simulink model "aes_impl_decrypt_smc"  (R2015b)
settings: Solver=FixedStepDiscrete  SolverMode=SingleTasking  StartTime=0.0  StopTime=1000e-6  RelTol=1e-3
undefined symbols (not defined in the file): a, b, input_sample_rate
libraries: shlslibv1 x3018
(part 8 of 20)

== system aes_impl_decrypt_smc/Round2/Subsystem8/Subsystem1 ==
  In1 : Inport
  In2 : Inport  Port=2
  In3 : Inport  Port=3
  In4 : Inport  Port=4
  Mixcolumn : Subsystem
  Mixcolumn1 : Subsystem
  Mixcolumn2 : Subsystem
  Mixcolumn3 : Subsystem
  Out1 : Outport
  Out2 : Outport  Port=2
  Out3 : Outport  Port=3
  Out4 : Outport  Port=4
  wires:
  Mixcolumn/1(Out1) -> Out1/1
  In4/1 -> Mixcolumn/4(In4), Mixcolumn1/4(In4), Mixcolumn2/4(In4), Mixcolumn3/4(In4)
  Mixcolumn2/1(Out1) -> Out3/1
  Mixcolumn1/1(Out1) -> Out2/1
  In2/1 -> Mixcolumn/2(In2), Mixcolumn1/2(In2), Mixcolumn3/2(In2), Mixcolumn2/2(In2)
  In1/1 -> Mixcolumn2/1(In1), Mixcolumn3/1(In1), Mixcolumn1/1(In1), Mixcolumn/1(In1)
  In3/1 -> Mixcolumn/3(In3), Mixcolumn1/3(In3), Mixcolumn3/3(In3), Mixcolumn2/3(In3)
  Mixcolumn3/1(Out1) -> Out4/1

== system aes_impl_decrypt_smc/Round2/Subsystem8/Subsystem2 ==
  In1 : Inport
  In2 : Inport  Port=2
  In3 : Inport  Port=3
  In4 : Inport  Port=4
  Mixcolumn : Subsystem
  Mixcolumn1 : Subsystem
  Mixcolumn2 : Subsystem
  Mixcolumn3 : Subsystem
  Out1 : Outport
  Out2 : Outport  Port=2
  Out3 : Outport  Port=3
  Out4 : Outport  Port=4
  wires:
  Mixcolumn/1(Out1) -> Out1/1
  In4/1 -> Mixcolumn/4(In4), Mixcolumn1/4(In4), Mixcolumn2/4(In4), Mixcolumn3/4(In4)
  Mixcolumn2/1(Out1) -> Out3/1
  Mixcolumn1/1(Out1) -> Out2/1
  In2/1 -> Mixcolumn/2(In2), Mixcolumn1/2(In2), Mixcolumn3/2(In2), Mixcolumn2/2(In2)
  In1/1 -> Mixcolumn2/1(In1), Mixcolumn3/1(In1), Mixcolumn1/1(In1), Mixcolumn/1(In1)
  In3/1 -> Mixcolumn/3(In3), Mixcolumn1/3(In3), Mixcolumn3/3(In3), Mixcolumn2/3(In3)
  Mixcolumn3/1(Out1) -> Out4/1

== system aes_impl_decrypt_smc/Round2/Subsystem8/Subsystem3 ==
  In1 : Inport
  In2 : Inport  Port=2
  In3 : Inport  Port=3
  In4 : Inport  Port=4
  Mixcolumn : Subsystem
  Mixcolumn1 : Subsystem
  Mixcolumn2 : Subsystem
  Mixcolumn3 : Subsystem
  Out1 : Outport
  Out2 : Outport  Port=2
  Out3 : Outport  Port=3
  Out4 : Outport  Port=4
  wires:
  Mixcolumn/1(Out1) -> Out1/1
  In4/1 -> Mixcolumn/4(In4), Mixcolumn1/4(In4), Mixcolumn2/4(In4), Mixcolumn3/4(In4)
  Mixcolumn2/1(Out1) -> Out3/1
  Mixcolumn1/1(Out1) -> Out2/1
  In2/1 -> Mixcolumn/2(In2), Mixcolumn1/2(In2), Mixcolumn3/2(In2), Mixcolumn2/2(In2)
  In1/1 -> Mixcolumn2/1(In1), Mixcolumn3/1(In1), Mixcolumn1/1(In1), Mixcolumn/1(In1)
  In3/1 -> Mixcolumn/3(In3), Mixcolumn1/3(In3), Mixcolumn3/3(In3), Mixcolumn2/3(In3)
  Mixcolumn3/1(Out1) -> Out4/1

== system aes_impl_decrypt_smc/Round2/Subsystem8/Subsystem4 ==
  In1 : Inport
  In2 : Inport  Port=2
  In3 : Inport  Port=3
  In4 : Inport  Port=4
  ROM{1..4} (4 alike) : shlslibv1/Memories/ROM  syn_rom_vec=sbox  syn_rom_auto_wl=on  syn_out_wl=8  syn_out_fl=0  syn_out_dt=unsigned  syn_out_sat=on  syn_out_rnd=on  syn_en_port=off  synBlockType=primitive  synLatency=1  synBlockId=62  syn_dual_port=off
  Out1 : Outport
  Out2 : Outport  Port=2
  Out3 : Outport  Port=3
  Out4 : Outport  Port=4
  wires:
  In1/1 -> ROM4/1
  In4/1 -> ROM3/1
  In3/1 -> ROM2/1
  ROM4/1 -> Out1/1
  ROM1/1 -> Out2/1
  ROM2/1 -> Out3/1
  ROM3/1 -> Out4/1
  In2/1 -> ROM1/1

== system aes_impl_decrypt_smc/Round2/Subsystem8/Subsystem5 ==
  In1 : Inport
  In2 : Inport  Port=2
  In3 : Inport  Port=3
  In4 : Inport  Port=4
  ROM{1..4} (4 alike) : shlslibv1/Memories/ROM  syn_rom_vec=sbox  syn_rom_auto_wl=on  syn_out_wl=8  syn_out_fl=0  syn_out_dt=unsigned  syn_out_sat=on  syn_out_rnd=on  syn_en_port=off  synBlockType=primitive  synLatency=1  synBlockId=62  syn_dual_port=off
  Out1 : Outport
  Out2 : Outport  Port=2
  Out3 : Outport  Port=3
  Out4 : Outport  Port=4
  wires:
  In1/1 -> ROM4/1
  In4/1 -> ROM3/1
  In3/1 -> ROM2/1
  ROM4/1 -> Out1/1
  ROM1/1 -> Out2/1
  ROM2/1 -> Out3/1
  ROM3/1 -> Out4/1
  In2/1 -> ROM1/1

== system aes_impl_decrypt_smc/Round2/Subsystem8/Subsystem6 ==
  In1 : Inport
  In2 : Inport  Port=2
  In3 : Inport  Port=3
  In4 : Inport  Port=4
  ROM{1..4} (4 alike) : shlslibv1/Memories/ROM  syn_rom_vec=sbox  syn_rom_auto_wl=on  syn_out_wl=8  syn_out_fl=0  syn_out_dt=unsigned  syn_out_sat=on  syn_out_rnd=on  syn_en_port=off  synBlockType=primitive  synLatency=1  synBlockId=62  syn_dual_port=off
  Out1 : Outport
  Out2 : Outport  Port=2
  Out3 : Outport  Port=3
  Out4 : Outport  Port=4
  wires:
  In1/1 -> ROM4/1
  In4/1 -> ROM3/1
  In3/1 -> ROM2/1
  ROM4/1 -> Out1/1
  ROM1/1 -> Out2/1
  ROM2/1 -> Out3/1
  ROM3/1 -> Out4/1
  In2/1 -> ROM1/1

== system aes_impl_decrypt_smc/Round2/Subsystem8/Subsystem7 ==
  In1 : Inport
  In2 : Inport  Port=2
  In3 : Inport  Port=3
  In4 : Inport  Port=4
  ROM{1..4} (4 alike) : shlslibv1/Memories/ROM  syn_rom_vec=sbox  syn_rom_auto_wl=on  syn_out_wl=8  syn_out_fl=0  syn_out_dt=unsigned  syn_out_sat=on  syn_out_rnd=on  syn_en_port=off  synBlockType=primitive  synLatency=1  synBlockId=62  syn_dual_port=off
  Out1 : Outport
  Out2 : Outport  Port=2
  Out3 : Outport  Port=3
  Out4 : Outport  Port=4
  wires:
  In1/1 -> ROM4/1
  In4/1 -> ROM3/1
  In3/1 -> ROM2/1
  ROM4/1 -> Out1/1
  ROM1/1 -> Out2/1
  ROM2/1 -> Out3/1
  ROM3/1 -> Out4/1
  In2/1 -> ROM1/1

== system aes_impl_decrypt_smc/Round20/Subsystem8/Subsystem ==
  In1 : Inport
  In2 : Inport  Port=2
  In3 : Inport  Port=3
  In4 : Inport  Port=4
  In5 : Inport  Port=5
  In6 : Inport  Port=6
  In7 : Inport  Port=7
  In8 : Inport  Port=8
  In9 : Inport  Port=9
  In10 : Inport  Port=10
  In11 : Inport  Port=11
  In12 : Inport  Port=12
  In13 : Inport  Port=13
  In14 : Inport  Port=14
  In15 : Inport  Port=15
  In16 : Inport  Port=16
  Out1 : Outport
  Out2 : Outport  Port=2
  Out3 : Outport  Port=3
  Out4 : Outport  Port=4
  Out5 : Outport  Port=5
  Out6 : Outport  Port=6
  Out7 : Outport  Port=7
  Out8 : Outport  Port=8
  Out9 : Outport  Port=9
  Out10 : Outport  Port=10
  Out11 : Outport  Port=11
  Out12 : Outport  Port=12
  Out13 : Outport  Port=13
  Out14 : Outport  Port=14
  Out15 : Outport  Port=15
  Out16 : Outport  Port=16
  wires:
  In1/1 -> Out1/1
  In5/1 -> Out5/1
  In9/1 -> Out9/1
  In13/1 -> Out13/1
  In2/1 -> Out6/1
  In3/1 -> Out11/1
  In4/1 -> Out16/1
  In6/1 -> Out10/1
  In7/1 -> Out15/1
  In8/1 -> Out4/1
  In10/1 -> Out14/1
  In11/1 -> Out3/1
  In12/1 -> Out8/1
  In14/1 -> Out2/1
  In15/1 -> Out7/1
  In16/1 -> Out12/1

== system aes_impl_decrypt_smc/Round20/Subsystem8/Subsystem1 ==
  In1 : Inport
  In2 : Inport  Port=2
  In3 : Inport  Port=3
  In4 : Inport  Port=4
  ROM{1..4} (4 alike) : shlslibv1/Memories/ROM  syn_rom_vec=isbox  syn_rom_auto_wl=on  syn_out_wl=8  syn_out_fl=0  syn_out_dt=unsigned  syn_out_sat=on  syn_out_rnd=on  syn_en_port=off  synBlockType=primitive  synLatency=1  synBlockId=62  syn_dual_port=off
  Out1 : Outport
  Out2 : Outport  Port=2
  Out3 : Outport  Port=3
  Out4 : Outport  Port=4
  wires:
  In1/1 -> ROM4/1
  In4/1 -> ROM3/1
  In3/1 -> ROM2/1
  ROM4/1 -> Out1/1
  ROM1/1 -> Out2/1
  ROM2/1 -> Out3/1
  ROM3/1 -> Out4/1
  In2/1 -> ROM1/1

== system aes_impl_decrypt_smc/Round20/Subsystem8/Subsystem2 ==
  In1 : Inport
  In2 : Inport  Port=2
  In3 : Inport  Port=3
  In4 : Inport  Port=4
  ROM{1..4} (4 alike) : shlslibv1/Memories/ROM  syn_rom_vec=isbox  syn_rom_auto_wl=on  syn_out_wl=8  syn_out_fl=0  syn_out_dt=unsigned  syn_out_sat=on  syn_out_rnd=on  syn_en_port=off  synBlockType=primitive  synLatency=1  synBlockId=62  syn_dual_port=off
  Out1 : Outport
  Out2 : Outport  Port=2
  Out3 : Outport  Port=3
  Out4 : Outport  Port=4
  wires:
  In1/1 -> ROM4/1
  In4/1 -> ROM3/1
  In3/1 -> ROM2/1
  ROM4/1 -> Out1/1
  ROM1/1 -> Out2/1
  ROM2/1 -> Out3/1
  ROM3/1 -> Out4/1
  In2/1 -> ROM1/1

== system aes_impl_decrypt_smc/Round20/Subsystem8/Subsystem3 ==
  In1 : Inport
  In2 : Inport  Port=2
  In3 : Inport  Port=3
  In4 : Inport  Port=4
  ROM{1..4} (4 alike) : shlslibv1/Memories/ROM  syn_rom_vec=isbox  syn_rom_auto_wl=on  syn_out_wl=8  syn_out_fl=0  syn_out_dt=unsigned  syn_out_sat=on  syn_out_rnd=on  syn_en_port=off  synBlockType=primitive  synLatency=1  synBlockId=62  syn_dual_port=off
  Out1 : Outport
  Out2 : Outport  Port=2
  Out3 : Outport  Port=3
  Out4 : Outport  Port=4
  wires:
  In1/1 -> ROM4/1
  In4/1 -> ROM3/1
  In3/1 -> ROM2/1
  ROM4/1 -> Out1/1
  ROM1/1 -> Out2/1
  ROM2/1 -> Out3/1
  ROM3/1 -> Out4/1
  In2/1 -> ROM1/1

== system aes_impl_decrypt_smc/Round20/Subsystem8/Subsystem4 ==
  In1 : Inport
  In2 : Inport  Port=2
  In3 : Inport  Port=3
  In4 : Inport  Port=4
  ROM{1..4} (4 alike) : shlslibv1/Memories/ROM  syn_rom_vec=isbox  syn_rom_auto_wl=on  syn_out_wl=8  syn_out_fl=0  syn_out_dt=unsigned  syn_out_sat=on  syn_out_rnd=on  syn_en_port=off  synBlockType=primitive  synLatency=1  synBlockId=62  syn_dual_port=off
  Out1 : Outport
  Out2 : Outport  Port=2
  Out3 : Outport  Port=3
  Out4 : Outport  Port=4
  wires:
  In1/1 -> ROM4/1
  In4/1 -> ROM3/1
  In3/1 -> ROM2/1
  ROM4/1 -> Out1/1
  ROM1/1 -> Out2/1
  ROM2/1 -> Out3/1
  ROM3/1 -> Out4/1
  In2/1 -> ROM1/1

== system aes_impl_decrypt_smc/Round20/Subsystem8/Subsystem5 ==
  In17 : Inport
  In18 : Inport  Port=2
  In19 : Inport  Port=3
  In20 : Inport  Port=4
  Mixcolumn : Subsystem
  Mixcolumn1 : Subsystem
  Mixcolumn2 : Subsystem
  Mixcolumn3 : Subsystem
  Out17 : Outport
  Out18 : Outport  Port=2
  Out19 : Outport  Port=3
  Out20 : Outport  Port=4
  wires:
  Mixcolumn3/1(Out1) -> Out20/1
  In20/1 -> Mixcolumn3/4(In4), Mixcolumn2/4(In4), Mixcolumn1/4(In4), Mixcolumn/4(In4)
  In17/1 -> Mixcolumn/1(In1), Mixcolumn1/1(In1), Mixcolumn3/1(In1), Mixcolumn2/1(In1)
  In19/1 -> Mixcolumn1/3(In3), Mixcolumn/3(In3), Mixcolumn3/3(In3), Mixcolumn2/3(In3)
  Mixcolumn1/1(Out1) -> Out18/1
  Mixcolumn/1(Out1) -> Out17/1
  In18/1 -> Mixcolumn1/2(In2), Mixcolumn/2(In2), Mixcolumn3/2(In2), Mixcolumn2/2(In2)
  Mixcolumn2/1(Out1) -> Out19/1

== system aes_impl_decrypt_smc/Round20/Subsystem8/Subsystem6 ==
  In17 : Inport
  In18 : Inport  Port=2
  In19 : Inport  Port=3
  In20 : Inport  Port=4
  Mixcolumn : Subsystem
  Mixcolumn1 : Subsystem
  Mixcolumn2 : Subsystem
  Mixcolumn3 : Subsystem
  Out17 : Outport
  Out18 : Outport  Port=2
  Out19 : Outport  Port=3
  Out20 : Outport  Port=4
  wires:
  Mixcolumn3/1(Out1) -> Out20/1
  In20/1 -> Mixcolumn3/4(In4), Mixcolumn2/4(In4), Mixcolumn1/4(In4), Mixcolumn/4(In4)
  In17/1 -> Mixcolumn/1(In1), Mixcolumn1/1(In1), Mixcolumn3/1(In1), Mixcolumn2/1(In1)
  In19/1 -> Mixcolumn1/3(In3), Mixcolumn/3(In3), Mixcolumn3/3(In3), Mixcolumn2/3(In3)
  Mixcolumn1/1(Out1) -> Out18/1
  Mixcolumn/1(Out1) -> Out17/1
  In18/1 -> Mixcolumn1/2(In2), Mixcolumn/2(In2), Mixcolumn3/2(In2), Mixcolumn2/2(In2)
  Mixcolumn2/1(Out1) -> Out19/1

== system aes_impl_decrypt_smc/Round20/Subsystem8/Subsystem7 ==
  In17 : Inport
  In18 : Inport  Port=2
  In19 : Inport  Port=3
  In20 : Inport  Port=4
  Mixcolumn : Subsystem
  Mixcolumn1 : Subsystem
  Mixcolumn2 : Subsystem
  Mixcolumn3 : Subsystem
  Out17 : Outport
  Out18 : Outport  Port=2
  Out19 : Outport  Port=3
  Out20 : Outport  Port=4
  wires:
  Mixcolumn3/1(Out1) -> Out20/1
  In20/1 -> Mixcolumn3/4(In4), Mixcolumn2/4(In4), Mixcolumn1/4(In4), Mixcolumn/4(In4)
  In17/1 -> Mixcolumn/1(In1), Mixcolumn1/1(In1), Mixcolumn3/1(In1), Mixcolumn2/1(In1)
  In19/1 -> Mixcolumn1/3(In3), Mixcolumn/3(In3), Mixcolumn3/3(In3), Mixcolumn2/3(In3)
  Mixcolumn1/1(Out1) -> Out18/1
  Mixcolumn/1(Out1) -> Out17/1
  In18/1 -> Mixcolumn1/2(In2), Mixcolumn/2(In2), Mixcolumn3/2(In2), Mixcolumn2/2(In2)
  Mixcolumn2/1(Out1) -> Out19/1

== system aes_impl_decrypt_smc/Round20/Subsystem8/Subsystem8 ==
  In17 : Inport
  In18 : Inport  Port=2
  In19 : Inport  Port=3
  In20 : Inport  Port=4
  Mixcolumn : Subsystem
  Mixcolumn1 : Subsystem
  Mixcolumn2 : Subsystem
  Mixcolumn3 : Subsystem
  Out17 : Outport
  Out18 : Outport  Port=2
  Out19 : Outport  Port=3
  Out20 : Outport  Port=4
  wires:
  Mixcolumn3/1(Out1) -> Out20/1
  In20/1 -> Mixcolumn3/4(In4), Mixcolumn2/4(In4), Mixcolumn1/4(In4), Mixcolumn/4(In4)
  In17/1 -> Mixcolumn/1(In1), Mixcolumn1/1(In1), Mixcolumn3/1(In1), Mixcolumn2/1(In1)
  In19/1 -> Mixcolumn1/3(In3), Mixcolumn/3(In3), Mixcolumn3/3(In3), Mixcolumn2/3(In3)
  Mixcolumn1/1(Out1) -> Out18/1
  Mixcolumn/1(Out1) -> Out17/1
  In18/1 -> Mixcolumn1/2(In2), Mixcolumn/2(In2), Mixcolumn3/2(In2), Mixcolumn2/2(In2)
  Mixcolumn2/1(Out1) -> Out19/1

== system aes_impl_decrypt_smc/Round3/Key1/Keygen1 ==
  In1 : Inport
  In2 : Inport  Port=2
  In3 : Inport  Port=3
  In4 : Inport  Port=4
  In5 : Inport  Port=5
  In6 : Inport  Port=6
  In7 : Inport  Port=7
  In8 : Inport  Port=8
  Binary Logic{,1..7} (8 alike) : shlslibv1/Math Functions/Binary Logic  syn_binlog_exp=a^b  synBlockType=primitive  synLatency=0  synBlockId=13
  Constant1 : shlslibv1/Sources/Constant  syn_cst_val=0  syn_cst_format=Specify  syn_cst_wl=8  syn_cst_fl=0  syn_cst_dt=unsigned  syn_cst_rnd=on  syn_cst_st=-1  synBlockType=primitive  synLatency=0  synBlockId=15
  Constant2 : shlslibv1/Sources/Constant  syn_cst_val=0  syn_cst_format=Specify  syn_cst_wl=8  syn_cst_fl=0  syn_cst_dt=unsigned  syn_cst_rnd=on  syn_cst_st=-1  synBlockType=primitive  synLatency=0  synBlockId=15
  Constant3 : shlslibv1/Sources/Constant  syn_cst_val=0  syn_cst_format=Specify  syn_cst_wl=8  syn_cst_fl=0  syn_cst_dt=unsigned  syn_cst_rnd=on  syn_cst_st=-1  synBlockType=primitive  synLatency=0  synBlockId=15
  Constant4 : shlslibv1/Sources/Constant  syn_cst_val=16  syn_cst_format=Specify  syn_cst_wl=8  syn_cst_fl=0  syn_cst_dt=unsigned  syn_cst_rnd=on  syn_cst_st=-1  synBlockType=primitive  synLatency=0  synBlockId=15
  Subsystem4 : Subsystem
  Out1 : Outport
  Out2 : Outport  Port=2
  Out3 : Outport  Port=3
  Out4 : Outport  Port=4
  wires:
  Constant1/1 -> Binary Logic3/2
  Binary Logic3/1 -> Out2/1
  Binary Logic5/1 -> Out3/1
  Binary Logic2/1 -> Out1/1
  Constant3/1 -> Binary Logic7/2
  Binary Logic7/1 -> Out4/1
  Constant2/1 -> Binary Logic5/2
  Subsystem4/3(Out3) -> Binary Logic4/2
  In7/1 -> Subsystem4/2(In2)
  In6/1 -> Subsystem4/1(In1)
  Subsystem4/4(Out4) -> Binary Logic6/2
  Subsystem4/2(Out2) -> Binary Logic1/2
  Subsystem4/1(Out1) -> Binary Logic/2
  In8/1 -> Subsystem4/3(In3)
  In5/1 -> Subsystem4/4(In4)
  In1/1 -> Binary Logic/1
  In2/1 -> Binary Logic1/1
  In3/1 -> Binary Logic4/1
  In4/1 -> Binary Logic6/1
  Constant4/1 -> Binary Logic2/2
  Binary Logic/1 -> Binary Logic2/1
  Binary Logic1/1 -> Binary Logic3/1
  Binary Logic4/1 -> Binary Logic5/1
  Binary Logic6/1 -> Binary Logic7/1

== system aes_impl_decrypt_smc/Round3/Key1/Keygen2 ==
  In1 : Inport
  In2 : Inport  Port=2
  In3 : Inport  Port=3
  In4 : Inport  Port=4
  In5 : Inport  Port=5
  In6 : Inport  Port=6
  In7 : Inport  Port=7
  In8 : Inport  Port=8
  Binary Logic{,1..3} (4 alike) : shlslibv1/Math Functions/Binary Logic  syn_binlog_exp=a^b  synBlockType=primitive  synLatency=0  synBlockId=13
  Out1 : Outport
  Out2 : Outport  Port=2
  Out3 : Outport  Port=3
  Out4 : Outport  Port=4
  wires:
  In6/1 -> Binary Logic1/2
  In2/1 -> Binary Logic1/1
  Binary Logic2/1 -> Out3/1
  In7/1 -> Binary Logic2/2
  In8/1 -> Binary Logic3/2
  Binary Logic1/1 -> Out2/1
  In3/1 -> Binary Logic2/1
  In4/1 -> Binary Logic3/1
  Binary Logic3/1 -> Out4/1
  In1/1 -> Binary Logic/1
  In5/1 -> Binary Logic/2
  Binary Logic/1 -> Out1/1

== system aes_impl_decrypt_smc/Round3/Key1/Keygen3 ==
  In1 : Inport
  In2 : Inport  Port=2
  In3 : Inport  Port=3
  In4 : Inport  Port=4
  In5 : Inport  Port=5
  In6 : Inport  Port=6
  In7 : Inport  Port=7
  In8 : Inport  Port=8
  Binary Logic{,1..3} (4 alike) : shlslibv1/Math Functions/Binary Logic  syn_binlog_exp=a^b  synBlockType=primitive  synLatency=0  synBlockId=13
  Out1 : Outport
  Out2 : Outport  Port=2
  Out3 : Outport  Port=3
  Out4 : Outport  Port=4
  wires:
  In6/1 -> Binary Logic1/2
  In2/1 -> Binary Logic1/1
  Binary Logic2/1 -> Out3/1
  In7/1 -> Binary Logic2/2
  In8/1 -> Binary Logic3/2
  Binary Logic1/1 -> Out2/1
  In3/1 -> Binary Logic2/1
  In4/1 -> Binary Logic3/1
  Binary Logic3/1 -> Out4/1
  In1/1 -> Binary Logic/1
  In5/1 -> Binary Logic/2
  Binary Logic/1 -> Out1/1

== system aes_impl_decrypt_smc/Round3/Key1/Keygen4 ==
  In1 : Inport
  In2 : Inport  Port=2
  In3 : Inport  Port=3
  In4 : Inport  Port=4
  In5 : Inport  Port=5
  In6 : Inport  Port=6
  In7 : Inport  Port=7
  In8 : Inport  Port=8
  Binary Logic{,1..3} (4 alike) : shlslibv1/Math Functions/Binary Logic  syn_binlog_exp=a^b  synBlockType=primitive  synLatency=0  synBlockId=13
  Out1 : Outport
  Out2 : Outport  Port=2
  Out3 : Outport  Port=3
  Out4 : Outport  Port=4
  wires:
  In6/1 -> Binary Logic1/2
  In2/1 -> Binary Logic1/1
  Binary Logic2/1 -> Out3/1
  In7/1 -> Binary Logic2/2
  In8/1 -> Binary Logic3/2
  Binary Logic1/1 -> Out2/1
  In3/1 -> Binary Logic2/1
  In4/1 -> Binary Logic3/1
  Binary Logic3/1 -> Out4/1
  In1/1 -> Binary Logic/1
  In5/1 -> Binary Logic/2
  Binary Logic/1 -> Out1/1

== system aes_impl_decrypt_smc/Round3/Subsystem8/Subsystem ==
  In1 : Inport
  In2 : Inport  Port=2
  In3 : Inport  Port=3
  In4 : Inport  Port=4
  Mixcolumn : Subsystem
  Mixcolumn1 : Subsystem
  Mixcolumn2 : Subsystem
  Mixcolumn3 : Subsystem
  Out1 : Outport
  Out2 : Outport  Port=2
  Out3 : Outport  Port=3
  Out4 : Outport  Port=4
  wires:
  Mixcolumn/1(Out1) -> Out1/1
  In4/1 -> Mixcolumn/4(In4), Mixcolumn1/4(In4), Mixcolumn2/4(In4), Mixcolumn3/4(In4)
  Mixcolumn2/1(Out1) -> Out3/1
  Mixcolumn1/1(Out1) -> Out2/1
  In2/1 -> Mixcolumn/2(In2), Mixcolumn1/2(In2), Mixcolumn3/2(In2), Mixcolumn2/2(In2)
  In1/1 -> Mixcolumn2/1(In1), Mixcolumn3/1(In1), Mixcolumn1/1(In1), Mixcolumn/1(In1)
  In3/1 -> Mixcolumn/3(In3), Mixcolumn1/3(In3), Mixcolumn3/3(In3), Mixcolumn2/3(In3)
  Mixcolumn3/1(Out1) -> Out4/1

== system aes_impl_decrypt_smc/Round3/Subsystem8/Subsystem1 ==
  In1 : Inport
  In2 : Inport  Port=2
  In3 : Inport  Port=3
  In4 : Inport  Port=4
  Mixcolumn : Subsystem
  Mixcolumn1 : Subsystem
  Mixcolumn2 : Subsystem
  Mixcolumn3 : Subsystem
  Out1 : Outport
  Out2 : Outport  Port=2
  Out3 : Outport  Port=3
  Out4 : Outport  Port=4
  wires:
  Mixcolumn/1(Out1) -> Out1/1
  In4/1 -> Mixcolumn/4(In4), Mixcolumn1/4(In4), Mixcolumn2/4(In4), Mixcolumn3/4(In4)
  Mixcolumn2/1(Out1) -> Out3/1
  Mixcolumn1/1(Out1) -> Out2/1
  In2/1 -> Mixcolumn/2(In2), Mixcolumn1/2(In2), Mixcolumn3/2(In2), Mixcolumn2/2(In2)
  In1/1 -> Mixcolumn2/1(In1), Mixcolumn3/1(In1), Mixcolumn1/1(In1), Mixcolumn/1(In1)
  In3/1 -> Mixcolumn/3(In3), Mixcolumn1/3(In3), Mixcolumn3/3(In3), Mixcolumn2/3(In3)
  Mixcolumn3/1(Out1) -> Out4/1

== system aes_impl_decrypt_smc/Round3/Subsystem8/Subsystem2 ==
  In1 : Inport
  In2 : Inport  Port=2
  In3 : Inport  Port=3
  In4 : Inport  Port=4
  Mixcolumn : Subsystem
  Mixcolumn1 : Subsystem
  Mixcolumn2 : Subsystem
  Mixcolumn3 : Subsystem
  Out1 : Outport
  Out2 : Outport  Port=2
  Out3 : Outport  Port=3
  Out4 : Outport  Port=4
  wires:
  Mixcolumn/1(Out1) -> Out1/1
  In4/1 -> Mixcolumn/4(In4), Mixcolumn1/4(In4), Mixcolumn2/4(In4), Mixcolumn3/4(In4)
  Mixcolumn2/1(Out1) -> Out3/1
  Mixcolumn1/1(Out1) -> Out2/1
  In2/1 -> Mixcolumn/2(In2), Mixcolumn1/2(In2), Mixcolumn3/2(In2), Mixcolumn2/2(In2)
  In1/1 -> Mixcolumn2/1(In1), Mixcolumn3/1(In1), Mixcolumn1/1(In1), Mixcolumn/1(In1)
  In3/1 -> Mixcolumn/3(In3), Mixcolumn1/3(In3), Mixcolumn3/3(In3), Mixcolumn2/3(In3)
  Mixcolumn3/1(Out1) -> Out4/1

== system aes_impl_decrypt_smc/Round3/Subsystem8/Subsystem3 ==
  In1 : Inport
  In2 : Inport  Port=2
  In3 : Inport  Port=3
  In4 : Inport  Port=4
  Mixcolumn : Subsystem
  Mixcolumn1 : Subsystem
  Mixcolumn2 : Subsystem
  Mixcolumn3 : Subsystem
  Out1 : Outport
  Out2 : Outport  Port=2
  Out3 : Outport  Port=3
  Out4 : Outport  Port=4
  wires:
  Mixcolumn/1(Out1) -> Out1/1
  In4/1 -> Mixcolumn/4(In4), Mixcolumn1/4(In4), Mixcolumn2/4(In4), Mixcolumn3/4(In4)
  Mixcolumn2/1(Out1) -> Out3/1
  Mixcolumn1/1(Out1) -> Out2/1
  In2/1 -> Mixcolumn/2(In2), Mixcolumn1/2(In2), Mixcolumn3/2(In2), Mixcolumn2/2(In2)
  In1/1 -> Mixcolumn2/1(In1), Mixcolumn3/1(In1), Mixcolumn1/1(In1), Mixcolumn/1(In1)
  In3/1 -> Mixcolumn/3(In3), Mixcolumn1/3(In3), Mixcolumn3/3(In3), Mixcolumn2/3(In3)
  Mixcolumn3/1(Out1) -> Out4/1

== system aes_impl_decrypt_smc/Round3/Subsystem8/Subsystem4 ==
  In1 : Inport
  In2 : Inport  Port=2
  In3 : Inport  Port=3
  In4 : Inport  Port=4
  ROM{1..4} (4 alike) : shlslibv1/Memories/ROM  syn_rom_vec=sbox  syn_rom_auto_wl=on  syn_out_wl=8  syn_out_fl=0  syn_out_dt=unsigned  syn_out_sat=on  syn_out_rnd=on  syn_en_port=off  synBlockType=primitive  synLatency=1  synBlockId=62  syn_dual_port=off
  Out1 : Outport
  Out2 : Outport  Port=2
  Out3 : Outport  Port=3
  Out4 : Outport  Port=4
  wires:
  In1/1 -> ROM4/1
  In4/1 -> ROM3/1
  In3/1 -> ROM2/1
  ROM4/1 -> Out1/1
  ROM1/1 -> Out2/1
  ROM2/1 -> Out3/1
  ROM3/1 -> Out4/1
  In2/1 -> ROM1/1

== system aes_impl_decrypt_smc/Round3/Subsystem8/Subsystem5 ==
  In1 : Inport
  In2 : Inport  Port=2
  In3 : Inport  Port=3
  In4 : Inport  Port=4
  ROM{1..4} (4 alike) : shlslibv1/Memories/ROM  syn_rom_vec=sbox  syn_rom_auto_wl=on  syn_out_wl=8  syn_out_fl=0  syn_out_dt=unsigned  syn_out_sat=on  syn_out_rnd=on  syn_en_port=off  synBlockType=primitive  synLatency=1  synBlockId=62  syn_dual_port=off
  Out1 : Outport
  Out2 : Outport  Port=2
  Out3 : Outport  Port=3
  Out4 : Outport  Port=4
  wires:
  In1/1 -> ROM4/1
  In4/1 -> ROM3/1
  In3/1 -> ROM2/1
  ROM4/1 -> Out1/1
  ROM1/1 -> Out2/1
  ROM2/1 -> Out3/1
  ROM3/1 -> Out4/1
  In2/1 -> ROM1/1

== system aes_impl_decrypt_smc/Round3/Subsystem8/Subsystem6 ==
  In1 : Inport
  In2 : Inport  Port=2
  In3 : Inport  Port=3
  In4 : Inport  Port=4
  ROM{1..4} (4 alike) : shlslibv1/Memories/ROM  syn_rom_vec=sbox  syn_rom_auto_wl=on  syn_out_wl=8  syn_out_fl=0  syn_out_dt=unsigned  syn_out_sat=on  syn_out_rnd=on  syn_en_port=off  synBlockType=primitive  synLatency=1  synBlockId=62  syn_dual_port=off
  Out1 : Outport
  Out2 : Outport  Port=2
  Out3 : Outport  Port=3
  Out4 : Outport  Port=4
  wires:
  In1/1 -> ROM4/1
  In4/1 -> ROM3/1
  In3/1 -> ROM2/1
  ROM4/1 -> Out1/1
  ROM1/1 -> Out2/1
  ROM2/1 -> Out3/1
  ROM3/1 -> Out4/1
  In2/1 -> ROM1/1

== system aes_impl_decrypt_smc/Round3/Subsystem8/Subsystem7 ==
  In1 : Inport
  In2 : Inport  Port=2
  In3 : Inport  Port=3
  In4 : Inport  Port=4
  ROM{1..4} (4 alike) : shlslibv1/Memories/ROM  syn_rom_vec=sbox  syn_rom_auto_wl=on  syn_out_wl=8  syn_out_fl=0  syn_out_dt=unsigned  syn_out_sat=on  syn_out_rnd=on  syn_en_port=off  synBlockType=primitive  synLatency=1  synBlockId=62  syn_dual_port=off
  Out1 : Outport
  Out2 : Outport  Port=2
  Out3 : Outport  Port=3
  Out4 : Outport  Port=4
  wires:
  In1/1 -> ROM4/1
  In4/1 -> ROM3/1
  In3/1 -> ROM2/1
  ROM4/1 -> Out1/1
  ROM1/1 -> Out2/1
  ROM2/1 -> Out3/1
  ROM3/1 -> Out4/1
  In2/1 -> ROM1/1

== system aes_impl_decrypt_smc/Round4/Key1/Keygen1 ==
  In1 : Inport
  In2 : Inport  Port=2
  In3 : Inport  Port=3
  In4 : Inport  Port=4
  In5 : Inport  Port=5
  In6 : Inport  Port=6
  In7 : Inport  Port=7
  In8 : Inport  Port=8
  Binary Logic{,1..7} (8 alike) : shlslibv1/Math Functions/Binary Logic  syn_binlog_exp=a^b  synBlockType=primitive  synLatency=0  synBlockId=13
  Constant1 : shlslibv1/Sources/Constant  syn_cst_val=0  syn_cst_format=Specify  syn_cst_wl=8  syn_cst_fl=0  syn_cst_dt=unsigned  syn_cst_rnd=on  syn_cst_st=-1  synBlockType=primitive  synLatency=0  synBlockId=15
  Constant2 : shlslibv1/Sources/Constant  syn_cst_val=0  syn_cst_format=Specify  syn_cst_wl=8  syn_cst_fl=0  syn_cst_dt=unsigned  syn_cst_rnd=on  syn_cst_st=-1  synBlockType=primitive  synLatency=0  synBlockId=15
  Constant3 : shlslibv1/Sources/Constant  syn_cst_val=0  syn_cst_format=Specify  syn_cst_wl=8  syn_cst_fl=0  syn_cst_dt=unsigned  syn_cst_rnd=on  syn_cst_st=-1  synBlockType=primitive  synLatency=0  synBlockId=15
  Constant4 : shlslibv1/Sources/Constant  syn_cst_val=4  syn_cst_format=Specify  syn_cst_wl=8  syn_cst_fl=0  syn_cst_dt=unsigned  syn_cst_rnd=on  syn_cst_st=-1  synBlockType=primitive  synLatency=0  synBlockId=15
  Subsystem4 : Subsystem
  Out1 : Outport
  Out2 : Outport  Port=2
  Out3 : Outport  Port=3
  Out4 : Outport  Port=4
  wires:
  Constant1/1 -> Binary Logic3/2
  Binary Logic3/1 -> Out2/1
  Binary Logic5/1 -> Out3/1
  Binary Logic2/1 -> Out1/1
  Constant3/1 -> Binary Logic7/2
  Binary Logic7/1 -> Out4/1
  Constant2/1 -> Binary Logic5/2
  Subsystem4/3(Out3) -> Binary Logic4/2
  In7/1 -> Subsystem4/2(In2)
  In6/1 -> Subsystem4/1(In1)
  Subsystem4/4(Out4) -> Binary Logic6/2
  Subsystem4/2(Out2) -> Binary Logic1/2
  Subsystem4/1(Out1) -> Binary Logic/2
  In8/1 -> Subsystem4/3(In3)
  In5/1 -> Subsystem4/4(In4)
  In1/1 -> Binary Logic/1
  In2/1 -> Binary Logic1/1
  In3/1 -> Binary Logic4/1
  In4/1 -> Binary Logic6/1
  Constant4/1 -> Binary Logic2/2
  Binary Logic/1 -> Binary Logic2/1
  Binary Logic1/1 -> Binary Logic3/1
  Binary Logic4/1 -> Binary Logic5/1
  Binary Logic6/1 -> Binary Logic7/1

== system aes_impl_decrypt_smc/Round4/Key1/Keygen2 ==
  In1 : Inport
  In2 : Inport  Port=2
  In3 : Inport  Port=3
  In4 : Inport  Port=4
  In5 : Inport  Port=5
  In6 : Inport  Port=6
  In7 : Inport  Port=7
  In8 : Inport  Port=8
  Binary Logic{,1..3} (4 alike) : shlslibv1/Math Functions/Binary Logic  syn_binlog_exp=a^b  synBlockType=primitive  synLatency=0  synBlockId=13
  Out1 : Outport
  Out2 : Outport  Port=2
  Out3 : Outport  Port=3
  Out4 : Outport  Port=4
  wires:
  In6/1 -> Binary Logic1/2
  In2/1 -> Binary Logic1/1
  Binary Logic2/1 -> Out3/1
  In7/1 -> Binary Logic2/2
  In8/1 -> Binary Logic3/2
  Binary Logic1/1 -> Out2/1
  In3/1 -> Binary Logic2/1
  In4/1 -> Binary Logic3/1
  Binary Logic3/1 -> Out4/1
  In1/1 -> Binary Logic/1
  In5/1 -> Binary Logic/2
  Binary Logic/1 -> Out1/1

== system aes_impl_decrypt_smc/Round4/Key1/Keygen3 ==
  In1 : Inport
  In2 : Inport  Port=2
  In3 : Inport  Port=3
  In4 : Inport  Port=4
  In5 : Inport  Port=5
  In6 : Inport  Port=6
  In7 : Inport  Port=7
  In8 : Inport  Port=8
  Binary Logic{,1..3} (4 alike) : shlslibv1/Math Functions/Binary Logic  syn_binlog_exp=a^b  synBlockType=primitive  synLatency=0  synBlockId=13
  Out1 : Outport
  Out2 : Outport  Port=2
  Out3 : Outport  Port=3
  Out4 : Outport  Port=4
  wires:
  In6/1 -> Binary Logic1/2
  In2/1 -> Binary Logic1/1
  Binary Logic2/1 -> Out3/1
  In7/1 -> Binary Logic2/2
  In8/1 -> Binary Logic3/2
  Binary Logic1/1 -> Out2/1
  In3/1 -> Binary Logic2/1
  In4/1 -> Binary Logic3/1
  Binary Logic3/1 -> Out4/1
  In1/1 -> Binary Logic/1
  In5/1 -> Binary Logic/2
  Binary Logic/1 -> Out1/1

== system aes_impl_decrypt_smc/Round4/Key1/Keygen4 ==
  In1 : Inport
  In2 : Inport  Port=2
  In3 : Inport  Port=3
  In4 : Inport  Port=4
  In5 : Inport  Port=5
  In6 : Inport  Port=6
  In7 : Inport  Port=7
  In8 : Inport  Port=8
  Binary Logic{,1..3} (4 alike) : shlslibv1/Math Functions/Binary Logic  syn_binlog_exp=a^b  synBlockType=primitive  synLatency=0  synBlockId=13
  Out1 : Outport
  Out2 : Outport  Port=2
  Out3 : Outport  Port=3
  Out4 : Outport  Port=4
  wires:
  In6/1 -> Binary Logic1/2
  In2/1 -> Binary Logic1/1
  Binary Logic2/1 -> Out3/1
  In7/1 -> Binary Logic2/2
  In8/1 -> Binary Logic3/2
  Binary Logic1/1 -> Out2/1
  In3/1 -> Binary Logic2/1
  In4/1 -> Binary Logic3/1
  Binary Logic3/1 -> Out4/1
  In1/1 -> Binary Logic/1
  In5/1 -> Binary Logic/2
  Binary Logic/1 -> Out1/1

== system aes_impl_decrypt_smc/Round4/Subsystem8/Subsystem ==
  In1 : Inport
  In2 : Inport  Port=2
  In3 : Inport  Port=3
  In4 : Inport  Port=4
  Mixcolumn : Subsystem
  Mixcolumn1 : Subsystem
  Mixcolumn2 : Subsystem
  Mixcolumn3 : Subsystem
  Out1 : Outport
  Out2 : Outport  Port=2
  Out3 : Outport  Port=3
  Out4 : Outport  Port=4
  wires:
  Mixcolumn/1(Out1) -> Out1/1
  In4/1 -> Mixcolumn/4(In4), Mixcolumn1/4(In4), Mixcolumn2/4(In4), Mixcolumn3/4(In4)
  Mixcolumn2/1(Out1) -> Out3/1
  Mixcolumn1/1(Out1) -> Out2/1
  In2/1 -> Mixcolumn/2(In2), Mixcolumn1/2(In2), Mixcolumn3/2(In2), Mixcolumn2/2(In2)
  In1/1 -> Mixcolumn2/1(In1), Mixcolumn3/1(In1), Mixcolumn1/1(In1), Mixcolumn/1(In1)
  In3/1 -> Mixcolumn/3(In3), Mixcolumn1/3(In3), Mixcolumn3/3(In3), Mixcolumn2/3(In3)
  Mixcolumn3/1(Out1) -> Out4/1

== system aes_impl_decrypt_smc/Round4/Subsystem8/Subsystem1 ==
  In1 : Inport
  In2 : Inport  Port=2
  In3 : Inport  Port=3
  In4 : Inport  Port=4
  Mixcolumn : Subsystem
  Mixcolumn1 : Subsystem
  Mixcolumn2 : Subsystem
  Mixcolumn3 : Subsystem
  Out1 : Outport
  Out2 : Outport  Port=2
  Out3 : Outport  Port=3
  Out4 : Outport  Port=4
  wires:
  Mixcolumn/1(Out1) -> Out1/1
  In4/1 -> Mixcolumn/4(In4), Mixcolumn1/4(In4), Mixcolumn2/4(In4), Mixcolumn3/4(In4)
  Mixcolumn2/1(Out1) -> Out3/1
  Mixcolumn1/1(Out1) -> Out2/1
  In2/1 -> Mixcolumn/2(In2), Mixcolumn1/2(In2), Mixcolumn3/2(In2), Mixcolumn2/2(In2)
  In1/1 -> Mixcolumn2/1(In1), Mixcolumn3/1(In1), Mixcolumn1/1(In1), Mixcolumn/1(In1)
  In3/1 -> Mixcolumn/3(In3), Mixcolumn1/3(In3), Mixcolumn3/3(In3), Mixcolumn2/3(In3)
  Mixcolumn3/1(Out1) -> Out4/1

== system aes_impl_decrypt_smc/Round4/Subsystem8/Subsystem2 ==
  In1 : Inport
  In2 : Inport  Port=2
  In3 : Inport  Port=3
  In4 : Inport  Port=4
  Mixcolumn : Subsystem
  Mixcolumn1 : Subsystem
  Mixcolumn2 : Subsystem
  Mixcolumn3 : Subsystem
  Out1 : Outport
  Out2 : Outport  Port=2
  Out3 : Outport  Port=3
  Out4 : Outport  Port=4
  wires:
  Mixcolumn/1(Out1) -> Out1/1
  In4/1 -> Mixcolumn/4(In4), Mixcolumn1/4(In4), Mixcolumn2/4(In4), Mixcolumn3/4(In4)
  Mixcolumn2/1(Out1) -> Out3/1
  Mixcolumn1/1(Out1) -> Out2/1
  In2/1 -> Mixcolumn/2(In2), Mixcolumn1/2(In2), Mixcolumn3/2(In2), Mixcolumn2/2(In2)
  In1/1 -> Mixcolumn2/1(In1), Mixcolumn3/1(In1), Mixcolumn1/1(In1), Mixcolumn/1(In1)
  In3/1 -> Mixcolumn/3(In3), Mixcolumn1/3(In3), Mixcolumn3/3(In3), Mixcolumn2/3(In3)
  Mixcolumn3/1(Out1) -> Out4/1

== system aes_impl_decrypt_smc/Round4/Subsystem8/Subsystem3 ==
  In1 : Inport
  In2 : Inport  Port=2
  In3 : Inport  Port=3
  In4 : Inport  Port=4
  Mixcolumn : Subsystem
  Mixcolumn1 : Subsystem
  Mixcolumn2 : Subsystem
  Mixcolumn3 : Subsystem
  Out1 : Outport
  Out2 : Outport  Port=2
  Out3 : Outport  Port=3
  Out4 : Outport  Port=4
  wires:
  Mixcolumn/1(Out1) -> Out1/1
  In4/1 -> Mixcolumn/4(In4), Mixcolumn1/4(In4), Mixcolumn2/4(In4), Mixcolumn3/4(In4)
  Mixcolumn2/1(Out1) -> Out3/1
  Mixcolumn1/1(Out1) -> Out2/1
  In2/1 -> Mixcolumn/2(In2), Mixcolumn1/2(In2), Mixcolumn3/2(In2), Mixcolumn2/2(In2)
  In1/1 -> Mixcolumn2/1(In1), Mixcolumn3/1(In1), Mixcolumn1/1(In1), Mixcolumn/1(In1)
  In3/1 -> Mixcolumn/3(In3), Mixcolumn1/3(In3), Mixcolumn3/3(In3), Mixcolumn2/3(In3)
  Mixcolumn3/1(Out1) -> Out4/1

== system aes_impl_decrypt_smc/Round4/Subsystem8/Subsystem4 ==
  In1 : Inport
  In2 : Inport  Port=2
  In3 : Inport  Port=3
  In4 : Inport  Port=4
  ROM{1..4} (4 alike) : shlslibv1/Memories/ROM  syn_rom_vec=sbox  syn_rom_auto_wl=on  syn_out_wl=8  syn_out_fl=0  syn_out_dt=unsigned  syn_out_sat=on  syn_out_rnd=on  syn_en_port=off  synBlockType=primitive  synLatency=1  synBlockId=62  syn_dual_port=off
  Out1 : Outport
  Out2 : Outport  Port=2
  Out3 : Outport  Port=3
  Out4 : Outport  Port=4
  wires:
  In1/1 -> ROM4/1
  In4/1 -> ROM3/1
  In3/1 -> ROM2/1
  ROM4/1 -> Out1/1
  ROM1/1 -> Out2/1
  ROM2/1 -> Out3/1
  ROM3/1 -> Out4/1
  In2/1 -> ROM1/1

== system aes_impl_decrypt_smc/Round4/Subsystem8/Subsystem5 ==
  In1 : Inport
  In2 : Inport  Port=2
  In3 : Inport  Port=3
  In4 : Inport  Port=4
  ROM{1..4} (4 alike) : shlslibv1/Memories/ROM  syn_rom_vec=sbox  syn_rom_auto_wl=on  syn_out_wl=8  syn_out_fl=0  syn_out_dt=unsigned  syn_out_sat=on  syn_out_rnd=on  syn_en_port=off  synBlockType=primitive  synLatency=1  synBlockId=62  syn_dual_port=off
  Out1 : Outport
  Out2 : Outport  Port=2
  Out3 : Outport  Port=3
  Out4 : Outport  Port=4
  wires:
  In1/1 -> ROM4/1
  In4/1 -> ROM3/1
  In3/1 -> ROM2/1
  ROM4/1 -> Out1/1
  ROM1/1 -> Out2/1
  ROM2/1 -> Out3/1
  ROM3/1 -> Out4/1
  In2/1 -> ROM1/1

== system aes_impl_decrypt_smc/Round4/Subsystem8/Subsystem6 ==
  In1 : Inport
  In2 : Inport  Port=2
  In3 : Inport  Port=3
  In4 : Inport  Port=4
  ROM{1..4} (4 alike) : shlslibv1/Memories/ROM  syn_rom_vec=sbox  syn_rom_auto_wl=on  syn_out_wl=8  syn_out_fl=0  syn_out_dt=unsigned  syn_out_sat=on  syn_out_rnd=on  syn_en_port=off  synBlockType=primitive  synLatency=1  synBlockId=62  syn_dual_port=off
  Out1 : Outport
  Out2 : Outport  Port=2
  Out3 : Outport  Port=3
  Out4 : Outport  Port=4
  wires:
  In1/1 -> ROM4/1
  In4/1 -> ROM3/1
  In3/1 -> ROM2/1
  ROM4/1 -> Out1/1
  ROM1/1 -> Out2/1
  ROM2/1 -> Out3/1
  ROM3/1 -> Out4/1
  In2/1 -> ROM1/1

== system aes_impl_decrypt_smc/Round4/Subsystem8/Subsystem7 ==
  In1 : Inport
  In2 : Inport  Port=2
  In3 : Inport  Port=3
  In4 : Inport  Port=4
  ROM{1..4} (4 alike) : shlslibv1/Memories/ROM  syn_rom_vec=sbox  syn_rom_auto_wl=on  syn_out_wl=8  syn_out_fl=0  syn_out_dt=unsigned  syn_out_sat=on  syn_out_rnd=on  syn_en_port=off  synBlockType=primitive  synLatency=1  synBlockId=62  syn_dual_port=off
  Out1 : Outport
  Out2 : Outport  Port=2
  Out3 : Outport  Port=3
  Out4 : Outport  Port=4
  wires:
  In1/1 -> ROM4/1
  In4/1 -> ROM3/1
  In3/1 -> ROM2/1
  ROM4/1 -> Out1/1
  ROM1/1 -> Out2/1
  ROM2/1 -> Out3/1
  ROM3/1 -> Out4/1
  In2/1 -> ROM1/1

== system aes_impl_decrypt_smc/Round5/Key1/Keygen1 ==
  In1 : Inport
  In2 : Inport  Port=2
  In3 : Inport  Port=3
  In4 : Inport  Port=4
  In5 : Inport  Port=5
  In6 : Inport  Port=6
  In7 : Inport  Port=7
  In8 : Inport  Port=8
  Binary Logic{,1..7} (8 alike) : shlslibv1/Math Functions/Binary Logic  syn_binlog_exp=a^b  synBlockType=primitive  synLatency=0  synBlockId=13
  Constant1 : shlslibv1/Sources/Constant  syn_cst_val=0  syn_cst_format=Specify  syn_cst_wl=8  syn_cst_fl=0  syn_cst_dt=unsigned  syn_cst_rnd=on  syn_cst_st=-1  synBlockType=primitive  synLatency=0  synBlockId=15
  Constant2 : shlslibv1/Sources/Constant  syn_cst_val=0  syn_cst_format=Specify  syn_cst_wl=8  syn_cst_fl=0  syn_cst_dt=unsigned  syn_cst_rnd=on  syn_cst_st=-1  synBlockType=primitive  synLatency=0  synBlockId=15
  Constant3 : shlslibv1/Sources/Constant  syn_cst_val=0  syn_cst_format=Specify  syn_cst_wl=8  syn_cst_fl=0  syn_cst_dt=unsigned  syn_cst_rnd=on  syn_cst_st=-1  synBlockType=primitive  synLatency=0  synBlockId=15
  Constant4 : shlslibv1/Sources/Constant  syn_cst_val=8  syn_cst_format=Specify  syn_cst_wl=8  syn_cst_fl=0  syn_cst_dt=unsigned  syn_cst_rnd=on  syn_cst_st=-1  synBlockType=primitive  synLatency=0  synBlockId=15
  Subsystem4 : Subsystem
  Out1 : Outport
  Out2 : Outport  Port=2
  Out3 : Outport  Port=3
  Out4 : Outport  Port=4
  wires:
  Constant1/1 -> Binary Logic3/2
  Binary Logic3/1 -> Out2/1
  Binary Logic5/1 -> Out3/1
  Binary Logic2/1 -> Out1/1
  Constant3/1 -> Binary Logic7/2
  Binary Logic7/1 -> Out4/1
  Constant2/1 -> Binary Logic5/2
  Subsystem4/3(Out3) -> Binary Logic4/2
  In7/1 -> Subsystem4/2(In2)
  In6/1 -> Subsystem4/1(In1)
  Subsystem4/4(Out4) -> Binary Logic6/2
  Subsystem4/2(Out2) -> Binary Logic1/2
  Subsystem4/1(Out1) -> Binary Logic/2
  In8/1 -> Subsystem4/3(In3)
  In5/1 -> Subsystem4/4(In4)
  In1/1 -> Binary Logic/1
  In2/1 -> Binary Logic1/1
  In3/1 -> Binary Logic4/1
  In4/1 -> Binary Logic6/1
  Constant4/1 -> Binary Logic2/2
  Binary Logic/1 -> Binary Logic2/1
  Binary Logic1/1 -> Binary Logic3/1
  Binary Logic4/1 -> Binary Logic5/1
  Binary Logic6/1 -> Binary Logic7/1

== system aes_impl_decrypt_smc/Round5/Key1/Keygen2 ==
  In1 : Inport
  In2 : Inport  Port=2
  In3 : Inport  Port=3
  In4 : Inport  Port=4
  In5 : Inport  Port=5
  In6 : Inport  Port=6
  In7 : Inport  Port=7
  In8 : Inport  Port=8
  Binary Logic{,1..3} (4 alike) : shlslibv1/Math Functions/Binary Logic  syn_binlog_exp=a^b  synBlockType=primitive  synLatency=0  synBlockId=13
  Out1 : Outport
  Out2 : Outport  Port=2
  Out3 : Outport  Port=3
  Out4 : Outport  Port=4
  wires:
  In6/1 -> Binary Logic1/2
  In2/1 -> Binary Logic1/1
  Binary Logic2/1 -> Out3/1
  In7/1 -> Binary Logic2/2
  In8/1 -> Binary Logic3/2
  Binary Logic1/1 -> Out2/1
  In3/1 -> Binary Logic2/1
  In4/1 -> Binary Logic3/1
  Binary Logic3/1 -> Out4/1
  In1/1 -> Binary Logic/1
  In5/1 -> Binary Logic/2
  Binary Logic/1 -> Out1/1

== system aes_impl_decrypt_smc/Round5/Key1/Keygen3 ==
  In1 : Inport
  In2 : Inport  Port=2
  In3 : Inport  Port=3
  In4 : Inport  Port=4
  In5 : Inport  Port=5
  In6 : Inport  Port=6
  In7 : Inport  Port=7
  In8 : Inport  Port=8
  Binary Logic{,1..3} (4 alike) : shlslibv1/Math Functions/Binary Logic  syn_binlog_exp=a^b  synBlockType=primitive  synLatency=0  synBlockId=13
  Out1 : Outport
  Out2 : Outport  Port=2
  Out3 : Outport  Port=3
  Out4 : Outport  Port=4
  wires:
  In6/1 -> Binary Logic1/2
  In2/1 -> Binary Logic1/1
  Binary Logic2/1 -> Out3/1
  In7/1 -> Binary Logic2/2
  In8/1 -> Binary Logic3/2
  Binary Logic1/1 -> Out2/1
  In3/1 -> Binary Logic2/1
  In4/1 -> Binary Logic3/1
  Binary Logic3/1 -> Out4/1
  In1/1 -> Binary Logic/1
  In5/1 -> Binary Logic/2
  Binary Logic/1 -> Out1/1

== system aes_impl_decrypt_smc/Round5/Key1/Keygen4 ==
  In1 : Inport
  In2 : Inport  Port=2
  In3 : Inport  Port=3
  In4 : Inport  Port=4
  In5 : Inport  Port=5
  In6 : Inport  Port=6
  In7 : Inport  Port=7
  In8 : Inport  Port=8
  Binary Logic{,1..3} (4 alike) : shlslibv1/Math Functions/Binary Logic  syn_binlog_exp=a^b  synBlockType=primitive  synLatency=0  synBlockId=13
  Out1 : Outport
  Out2 : Outport  Port=2
  Out3 : Outport  Port=3
  Out4 : Outport  Port=4
  wires:
  In6/1 -> Binary Logic1/2
  In2/1 -> Binary Logic1/1
  Binary Logic2/1 -> Out3/1
  In7/1 -> Binary Logic2/2
  In8/1 -> Binary Logic3/2
  Binary Logic1/1 -> Out2/1
  In3/1 -> Binary Logic2/1
  In4/1 -> Binary Logic3/1
  Binary Logic3/1 -> Out4/1
  In1/1 -> Binary Logic/1
  In5/1 -> Binary Logic/2
  Binary Logic/1 -> Out1/1

== system aes_impl_decrypt_smc/Round5/Subsystem8/Subsystem ==
  In1 : Inport
  In2 : Inport  Port=2
  In3 : Inport  Port=3
  In4 : Inport  Port=4
  Mixcolumn : Subsystem
  Mixcolumn1 : Subsystem
  Mixcolumn2 : Subsystem
  Mixcolumn3 : Subsystem
  Out1 : Outport
  Out2 : Outport  Port=2
  Out3 : Outport  Port=3
  Out4 : Outport  Port=4
  wires:
  Mixcolumn/1(Out1) -> Out1/1
  In4/1 -> Mixcolumn/4(In4), Mixcolumn1/4(In4), Mixcolumn2/4(In4), Mixcolumn3/4(In4)
  Mixcolumn2/1(Out1) -> Out3/1
  Mixcolumn1/1(Out1) -> Out2/1
  In2/1 -> Mixcolumn/2(In2), Mixcolumn1/2(In2), Mixcolumn3/2(In2), Mixcolumn2/2(In2)
  In1/1 -> Mixcolumn2/1(In1), Mixcolumn3/1(In1), Mixcolumn1/1(In1), Mixcolumn/1(In1)
  In3/1 -> Mixcolumn/3(In3), Mixcolumn1/3(In3), Mixcolumn3/3(In3), Mixcolumn2/3(In3)
  Mixcolumn3/1(Out1) -> Out4/1

== system aes_impl_decrypt_smc/Round5/Subsystem8/Subsystem1 ==
  In1 : Inport
  In2 : Inport  Port=2
  In3 : Inport  Port=3
  In4 : Inport  Port=4
  Mixcolumn : Subsystem
  Mixcolumn1 : Subsystem
  Mixcolumn2 : Subsystem
  Mixcolumn3 : Subsystem
  Out1 : Outport
  Out2 : Outport  Port=2
  Out3 : Outport  Port=3
  Out4 : Outport  Port=4
  wires:
  Mixcolumn/1(Out1) -> Out1/1
  In4/1 -> Mixcolumn/4(In4), Mixcolumn1/4(In4), Mixcolumn2/4(In4), Mixcolumn3/4(In4)
  Mixcolumn2/1(Out1) -> Out3/1
  Mixcolumn1/1(Out1) -> Out2/1
  In2/1 -> Mixcolumn/2(In2), Mixcolumn1/2(In2), Mixcolumn3/2(In2), Mixcolumn2/2(In2)
  In1/1 -> Mixcolumn2/1(In1), Mixcolumn3/1(In1), Mixcolumn1/1(In1), Mixcolumn/1(In1)
  In3/1 -> Mixcolumn/3(In3), Mixcolumn1/3(In3), Mixcolumn3/3(In3), Mixcolumn2/3(In3)
  Mixcolumn3/1(Out1) -> Out4/1

== system aes_impl_decrypt_smc/Round5/Subsystem8/Subsystem2 ==
  In1 : Inport
  In2 : Inport  Port=2
  In3 : Inport  Port=3
  In4 : Inport  Port=4
  Mixcolumn : Subsystem
  Mixcolumn1 : Subsystem
  Mixcolumn2 : Subsystem
  Mixcolumn3 : Subsystem
  Out1 : Outport
  Out2 : Outport  Port=2
  Out3 : Outport  Port=3
  Out4 : Outport  Port=4
  wires:
  Mixcolumn/1(Out1) -> Out1/1
  In4/1 -> Mixcolumn/4(In4), Mixcolumn1/4(In4), Mixcolumn2/4(In4), Mixcolumn3/4(In4)
  Mixcolumn2/1(Out1) -> Out3/1
  Mixcolumn1/1(Out1) -> Out2/1
  In2/1 -> Mixcolumn/2(In2), Mixcolumn1/2(In2), Mixcolumn3/2(In2), Mixcolumn2/2(In2)
  In1/1 -> Mixcolumn2/1(In1), Mixcolumn3/1(In1), Mixcolumn1/1(In1), Mixcolumn/1(In1)
  In3/1 -> Mixcolumn/3(In3), Mixcolumn1/3(In3), Mixcolumn3/3(In3), Mixcolumn2/3(In3)
  Mixcolumn3/1(Out1) -> Out4/1

== system aes_impl_decrypt_smc/Round5/Subsystem8/Subsystem3 ==
  In1 : Inport
  In2 : Inport  Port=2
  In3 : Inport  Port=3
  In4 : Inport  Port=4
  Mixcolumn : Subsystem
  Mixcolumn1 : Subsystem
  Mixcolumn2 : Subsystem
  Mixcolumn3 : Subsystem
  Out1 : Outport
  Out2 : Outport  Port=2
  Out3 : Outport  Port=3
  Out4 : Outport  Port=4
  wires:
  Mixcolumn/1(Out1) -> Out1/1
  In4/1 -> Mixcolumn/4(In4), Mixcolumn1/4(In4), Mixcolumn2/4(In4), Mixcolumn3/4(In4)
  Mixcolumn2/1(Out1) -> Out3/1
  Mixcolumn1/1(Out1) -> Out2/1
  In2/1 -> Mixcolumn/2(In2), Mixcolumn1/2(In2), Mixcolumn3/2(In2), Mixcolumn2/2(In2)
  In1/1 -> Mixcolumn2/1(In1), Mixcolumn3/1(In1), Mixcolumn1/1(In1), Mixcolumn/1(In1)
  In3/1 -> Mixcolumn/3(In3), Mixcolumn1/3(In3), Mixcolumn3/3(In3), Mixcolumn2/3(In3)
  Mixcolumn3/1(Out1) -> Out4/1

== system aes_impl_decrypt_smc/Round5/Subsystem8/Subsystem4 ==
  In1 : Inport
  In2 : Inport  Port=2
  In3 : Inport  Port=3
  In4 : Inport  Port=4
  ROM{1..4} (4 alike) : shlslibv1/Memories/ROM  syn_rom_vec=sbox  syn_rom_auto_wl=on  syn_out_wl=8  syn_out_fl=0  syn_out_dt=unsigned  syn_out_sat=on  syn_out_rnd=on  syn_en_port=off  synBlockType=primitive  synLatency=1  synBlockId=62  syn_dual_port=off
  Out1 : Outport
  Out2 : Outport  Port=2
  Out3 : Outport  Port=3
  Out4 : Outport  Port=4
  wires:
  In1/1 -> ROM4/1
  In4/1 -> ROM3/1
  In3/1 -> ROM2/1
  ROM4/1 -> Out1/1
  ROM1/1 -> Out2/1
  ROM2/1 -> Out3/1
  ROM3/1 -> Out4/1
  In2/1 -> ROM1/1

== system aes_impl_decrypt_smc/Round5/Subsystem8/Subsystem5 ==
  In1 : Inport
  In2 : Inport  Port=2
  In3 : Inport  Port=3
  In4 : Inport  Port=4
  ROM{1..4} (4 alike) : shlslibv1/Memories/ROM  syn_rom_vec=sbox  syn_rom_auto_wl=on  syn_out_wl=8  syn_out_fl=0  syn_out_dt=unsigned  syn_out_sat=on  syn_out_rnd=on  syn_en_port=off  synBlockType=primitive  synLatency=1  synBlockId=62  syn_dual_port=off
  Out1 : Outport
  Out2 : Outport  Port=2
  Out3 : Outport  Port=3
  Out4 : Outport  Port=4
  wires:
  In1/1 -> ROM4/1
  In4/1 -> ROM3/1
  In3/1 -> ROM2/1
  ROM4/1 -> Out1/1
  ROM1/1 -> Out2/1
  ROM2/1 -> Out3/1
  ROM3/1 -> Out4/1
  In2/1 -> ROM1/1

== system aes_impl_decrypt_smc/Round5/Subsystem8/Subsystem6 ==
  In1 : Inport
  In2 : Inport  Port=2
  In3 : Inport  Port=3
  In4 : Inport  Port=4
  ROM{1..4} (4 alike) : shlslibv1/Memories/ROM  syn_rom_vec=sbox  syn_rom_auto_wl=on  syn_out_wl=8  syn_out_fl=0  syn_out_dt=unsigned  syn_out_sat=on  syn_out_rnd=on  syn_en_port=off  synBlockType=primitive  synLatency=1  synBlockId=62  syn_dual_port=off
  Out1 : Outport
  Out2 : Outport  Port=2
  Out3 : Outport  Port=3
  Out4 : Outport  Port=4
  wires:
  In1/1 -> ROM4/1
  In4/1 -> ROM3/1
  In3/1 -> ROM2/1
  ROM4/1 -> Out1/1
  ROM1/1 -> Out2/1
  ROM2/1 -> Out3/1
  ROM3/1 -> Out4/1
  In2/1 -> ROM1/1

== system aes_impl_decrypt_smc/Round5/Subsystem8/Subsystem7 ==
  In1 : Inport
  In2 : Inport  Port=2
  In3 : Inport  Port=3
  In4 : Inport  Port=4
  ROM{1..4} (4 alike) : shlslibv1/Memories/ROM  syn_rom_vec=sbox  syn_rom_auto_wl=on  syn_out_wl=8  syn_out_fl=0  syn_out_dt=unsigned  syn_out_sat=on  syn_out_rnd=on  syn_en_port=off  synBlockType=primitive  synLatency=1  synBlockId=62  syn_dual_port=off
  Out1 : Outport
  Out2 : Outport  Port=2
  Out3 : Outport  Port=3
  Out4 : Outport  Port=4
  wires:
  In1/1 -> ROM4/1
  In4/1 -> ROM3/1
  In3/1 -> ROM2/1
  ROM4/1 -> Out1/1
  ROM1/1 -> Out2/1
  ROM2/1 -> Out3/1
  ROM3/1 -> Out4/1
  In2/1 -> ROM1/1

== system aes_impl_decrypt_smc/Round6/Key1/Keygen1 ==
  In1 : Inport
  In2 : Inport  Port=2
  In3 : Inport  Port=3
  In4 : Inport  Port=4
  In5 : Inport  Port=5
  In6 : Inport  Port=6
  In7 : Inport  Port=7
  In8 : Inport  Port=8
  Binary Logic{,1..7} (8 alike) : shlslibv1/Math Functions/Binary Logic  syn_binlog_exp=a^b  synBlockType=primitive  synLatency=0  synBlockId=13
  Constant1 : shlslibv1/Sources/Constant  syn_cst_val=0  syn_cst_format=Specify  syn_cst_wl=8  syn_cst_fl=0  syn_cst_dt=unsigned  syn_cst_rnd=on  syn_cst_st=-1  synBlockType=primitive  synLatency=0  synBlockId=15
  Constant2 : shlslibv1/Sources/Constant  syn_cst_val=0  syn_cst_format=Specify  syn_cst_wl=8  syn_cst_fl=0  syn_cst_dt=unsigned  syn_cst_rnd=on  syn_cst_st=-1  synBlockType=primitive  synLatency=0  synBlockId=15
  Constant3 : shlslibv1/Sources/Constant  syn_cst_val=0  syn_cst_format=Specify  syn_cst_wl=8  syn_cst_fl=0  syn_cst_dt=unsigned  syn_cst_rnd=on  syn_cst_st=-1  synBlockType=primitive  synLatency=0  synBlockId=15
  Constant4 : shlslibv1/Sources/Constant  syn_cst_val=32  syn_cst_format=Specify  syn_cst_wl=8  syn_cst_fl=0  syn_cst_dt=unsigned  syn_cst_rnd=on  syn_cst_st=-1  synBlockType=primitive  synLatency=0  synBlockId=15
  Subsystem4 : Subsystem
  Out1 : Outport
  Out2 : Outport  Port=2
  Out3 : Outport  Port=3
  Out4 : Outport  Port=4
  wires:
  Constant1/1 -> Binary Logic3/2
  Binary Logic3/1 -> Out2/1
  Binary Logic5/1 -> Out3/1
  Binary Logic2/1 -> Out1/1
  Constant3/1 -> Binary Logic7/2
  Binary Logic7/1 -> Out4/1
  Constant2/1 -> Binary Logic5/2
  Subsystem4/3(Out3) -> Binary Logic4/2
  In7/1 -> Subsystem4/2(In2)
  In6/1 -> Subsystem4/1(In1)
  Subsystem4/4(Out4) -> Binary Logic6/2
  Subsystem4/2(Out2) -> Binary Logic1/2
  Subsystem4/1(Out1) -> Binary Logic/2
  In8/1 -> Subsystem4/3(In3)
  In5/1 -> Subsystem4/4(In4)
  In1/1 -> Binary Logic/1
  In2/1 -> Binary Logic1/1
  In3/1 -> Binary Logic4/1
  In4/1 -> Binary Logic6/1
  Constant4/1 -> Binary Logic2/2
  Binary Logic/1 -> Binary Logic2/1
  Binary Logic1/1 -> Binary Logic3/1
  Binary Logic4/1 -> Binary Logic5/1
  Binary Logic6/1 -> Binary Logic7/1

== system aes_impl_decrypt_smc/Round6/Key1/Keygen2 ==
  In1 : Inport
  In2 : Inport  Port=2
  In3 : Inport  Port=3
  In4 : Inport  Port=4
  In5 : Inport  Port=5
  In6 : Inport  Port=6
  In7 : Inport  Port=7
  In8 : Inport  Port=8
  Binary Logic{,1..3} (4 alike) : shlslibv1/Math Functions/Binary Logic  syn_binlog_exp=a^b  synBlockType=primitive  synLatency=0  synBlockId=13
  Out1 : Outport
  Out2 : Outport  Port=2
  Out3 : Outport  Port=3
  Out4 : Outport  Port=4
  wires:
  In6/1 -> Binary Logic1/2
  In2/1 -> Binary Logic1/1
  Binary Logic2/1 -> Out3/1
  In7/1 -> Binary Logic2/2
  In8/1 -> Binary Logic3/2
  Binary Logic1/1 -> Out2/1
  In3/1 -> Binary Logic2/1
  In4/1 -> Binary Logic3/1
  Binary Logic3/1 -> Out4/1
  In1/1 -> Binary Logic/1
  In5/1 -> Binary Logic/2
  Binary Logic/1 -> Out1/1

== system aes_impl_decrypt_smc/Round6/Key1/Keygen3 ==
  In1 : Inport
  In2 : Inport  Port=2
  In3 : Inport  Port=3
  In4 : Inport  Port=4
  In5 : Inport  Port=5
  In6 : Inport  Port=6
  In7 : Inport  Port=7
  In8 : Inport  Port=8
  Binary Logic{,1..3} (4 alike) : shlslibv1/Math Functions/Binary Logic  syn_binlog_exp=a^b  synBlockType=primitive  synLatency=0  synBlockId=13
  Out1 : Outport
  Out2 : Outport  Port=2
  Out3 : Outport  Port=3
  Out4 : Outport  Port=4
  wires:
  In6/1 -> Binary Logic1/2
  In2/1 -> Binary Logic1/1
  Binary Logic2/1 -> Out3/1
  In7/1 -> Binary Logic2/2
  In8/1 -> Binary Logic3/2
  Binary Logic1/1 -> Out2/1
  In3/1 -> Binary Logic2/1
  In4/1 -> Binary Logic3/1
  Binary Logic3/1 -> Out4/1
  In1/1 -> Binary Logic/1
  In5/1 -> Binary Logic/2
  Binary Logic/1 -> Out1/1

== system aes_impl_decrypt_smc/Round6/Key1/Keygen4 ==
  In1 : Inport
  In2 : Inport  Port=2
  In3 : Inport  Port=3
  In4 : Inport  Port=4
  In5 : Inport  Port=5
  In6 : Inport  Port=6
  In7 : Inport  Port=7
  In8 : Inport  Port=8
  Binary Logic{,1..3} (4 alike) : shlslibv1/Math Functions/Binary Logic  syn_binlog_exp=a^b  synBlockType=primitive  synLatency=0  synBlockId=13
  Out1 : Outport
  Out2 : Outport  Port=2
  Out3 : Outport  Port=3
  Out4 : Outport  Port=4
  wires:
  In6/1 -> Binary Logic1/2
  In2/1 -> Binary Logic1/1
  Binary Logic2/1 -> Out3/1
  In7/1 -> Binary Logic2/2
  In8/1 -> Binary Logic3/2
  Binary Logic1/1 -> Out2/1
  In3/1 -> Binary Logic2/1
  In4/1 -> Binary Logic3/1
  Binary Logic3/1 -> Out4/1
  In1/1 -> Binary Logic/1
  In5/1 -> Binary Logic/2
  Binary Logic/1 -> Out1/1

== system aes_impl_decrypt_smc/Round6/Subsystem8/Subsystem ==
  In1 : Inport
  In2 : Inport  Port=2
  In3 : Inport  Port=3
  In4 : Inport  Port=4
  Mixcolumn : Subsystem
  Mixcolumn1 : Subsystem
  Mixcolumn2 : Subsystem
  Mixcolumn3 : Subsystem
  Out1 : Outport
  Out2 : Outport  Port=2
  Out3 : Outport  Port=3
  Out4 : Outport  Port=4
  wires:
  Mixcolumn/1(Out1) -> Out1/1
  In4/1 -> Mixcolumn/4(In4), Mixcolumn1/4(In4), Mixcolumn2/4(In4), Mixcolumn3/4(In4)
  Mixcolumn2/1(Out1) -> Out3/1
  Mixcolumn1/1(Out1) -> Out2/1
  In2/1 -> Mixcolumn/2(In2), Mixcolumn1/2(In2), Mixcolumn3/2(In2), Mixcolumn2/2(In2)
  In1/1 -> Mixcolumn2/1(In1), Mixcolumn3/1(In1), Mixcolumn1/1(In1), Mixcolumn/1(In1)
  In3/1 -> Mixcolumn/3(In3), Mixcolumn1/3(In3), Mixcolumn3/3(In3), Mixcolumn2/3(In3)
  Mixcolumn3/1(Out1) -> Out4/1

== system aes_impl_decrypt_smc/Round6/Subsystem8/Subsystem1 ==
  In1 : Inport
  In2 : Inport  Port=2
  In3 : Inport  Port=3
  In4 : Inport  Port=4
  Mixcolumn : Subsystem
  Mixcolumn1 : Subsystem
  Mixcolumn2 : Subsystem
  Mixcolumn3 : Subsystem
  Out1 : Outport
  Out2 : Outport  Port=2
  Out3 : Outport  Port=3
  Out4 : Outport  Port=4
  wires:
  Mixcolumn/1(Out1) -> Out1/1
  In4/1 -> Mixcolumn/4(In4), Mixcolumn1/4(In4), Mixcolumn2/4(In4), Mixcolumn3/4(In4)
  Mixcolumn2/1(Out1) -> Out3/1
  Mixcolumn1/1(Out1) -> Out2/1
  In2/1 -> Mixcolumn/2(In2), Mixcolumn1/2(In2), Mixcolumn3/2(In2), Mixcolumn2/2(In2)
  In1/1 -> Mixcolumn2/1(In1), Mixcolumn3/1(In1), Mixcolumn1/1(In1), Mixcolumn/1(In1)
  In3/1 -> Mixcolumn/3(In3), Mixcolumn1/3(In3), Mixcolumn3/3(In3), Mixcolumn2/3(In3)
  Mixcolumn3/1(Out1) -> Out4/1
